simulink model "facsimile_encoding"  (R2016a)
settings: Solver=VariableStepAuto  StartTime=0.0  StopTime=sim_time  RelTol=1e-3
PreLoadFcn:
  | if exist('loadData')
  |     loadData
  | end
StopFcn:
  | if exist('processOutput')
  |     processOutput
  | end
libraries: xbsIndex_r4 x25
settings Model: Creator=hieut  LastModifiedBy=hieut

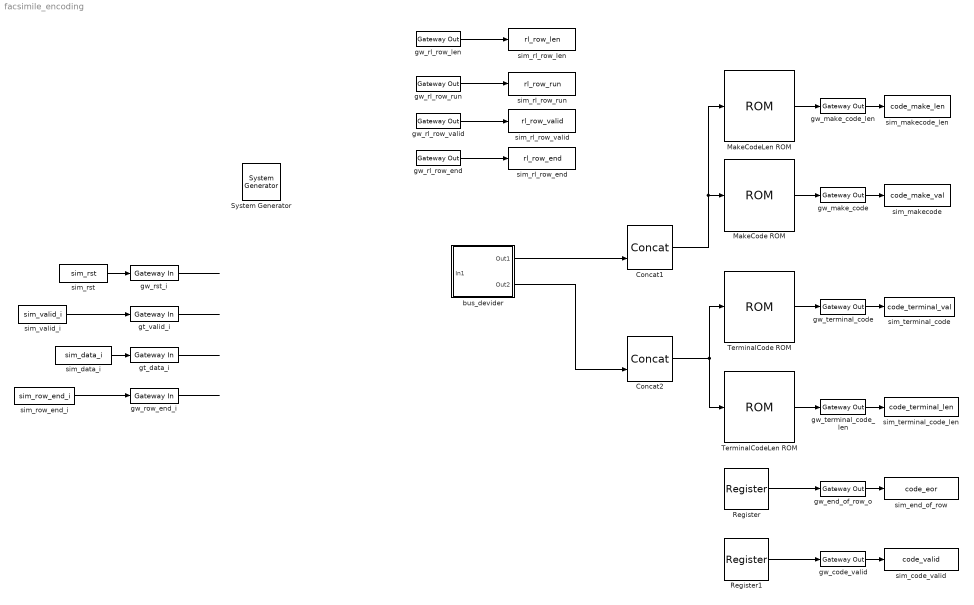
== system facsimile_encoding ==
  " System Generator" : xbsIndex_r4/ System Generator  Tag=genX  xilinxfamily=zynq  part=xc7z010  speed=-1  package=clg400  synthesis_tool=Vivado  clock_wrapper=Clock Enables  directory=./netlist  proj_type=Vivado  Synth_file=Vivado Synthesis Defaults  Impl_file=Vivado Implementation Defaults  testbench=off  simulink_period=1  sysclk_period=10  dcm_input_clock_period=10  incr_netlist=off  trim_vbits=Everywhere in SubSystem  dbl_ovrd=According to Block Masks  core_generation=According to Block Masks  run_coregen=off  deprecated_control=off  eval_field=0  block_type=sysgen
  Concat1 : xbsIndex_r4/Concat  num_inputs=2  dbl_ovrd=off  block_type=concat
  Concat2 : xbsIndex_r4/Concat  num_inputs=2  dbl_ovrd=off  block_type=concat
  MakeCode ROM : xbsIndex_r4/ROM  depth=64  initVector=rom_make_code_values  distributed_mem=Block RAM  rst=off  init_reg=0  en=off  latency=1  gui_display_data_type=Fixed-point  arith_type=Unsigned  n_bits=13  bin_pt=0  preci_type=Single  exp_width=8  frac_width=24  optimize=Area  use_rpm=on  dbl_ovrd=off  block_type=sprom
  MakeCodeLen ROM : xbsIndex_r4/ROM  depth=64  initVector=rom_make_code_lens  distributed_mem=Block RAM  rst=off  init_reg=0  en=off  latency=1  gui_display_data_type=Fixed-point  arith_type=Unsigned  n_bits=13  bin_pt=0  preci_type=Single  exp_width=8  frac_width=24  optimize=Area  use_rpm=on  dbl_ovrd=off  block_type=sprom
  Register : xbsIndex_r4/Register  init=0  rst=off  en=off  dbl_ovrd=off  block_type=register
  Register1 : xbsIndex_r4/Register  init=0  rst=off  en=off  dbl_ovrd=off  block_type=register
  TerminalCode ROM : xbsIndex_r4/ROM  depth=128  initVector=rom_terminal_code_values  distributed_mem=Block RAM  rst=off  init_reg=0  en=off  latency=1  gui_display_data_type=Fixed-point  arith_type=Unsigned  n_bits=13  bin_pt=0  preci_type=Single  exp_width=8  frac_width=24  optimize=Area  use_rpm=on  dbl_ovrd=off  block_type=sprom
  TerminalCodeLen ROM : xbsIndex_r4/ROM  depth=128  initVector=rom_terminal_code_lens  distributed_mem=Block RAM  rst=off  init_reg=0  en=off  latency=1  gui_display_data_type=Fixed-point  arith_type=Unsigned  n_bits=13  bin_pt=0  preci_type=Single  exp_width=8  frac_width=24  optimize=Area  use_rpm=on  dbl_ovrd=off  block_type=sprom
  bus_devider : Subsystem
  gt_data_i : xbsIndex_r4/Gateway In  gui_display_data_type=Boolean  arith_type=Boolean  n_bits=16  bin_pt=14  preci_type=Single  exp_width=8  frac_width=24  rows=1  columns=1  quantization="Round  (unbiased: +/- Inf)"  overflow=Saturate  period=1  UseAsADC=off  ADCChannel='1'  interface=None  automatic_assignment=on  address_offset=hex2dec('00')  intf_name=''  intf_description=''  default_value=0  timing_constraint=None  locs_specified=off  LOCs={}  io_standard={}  inherit_from_input=off  hdl_port=on  dbl_ovrd=off  block_type=gatewayin
  gt_valid_i : xbsIndex_r4/Gateway In  gui_display_data_type=Boolean  arith_type=Boolean  n_bits=16  bin_pt=14  preci_type=Single  exp_width=8  frac_width=24  rows=1  columns=1  quantization="Round  (unbiased: +/- Inf)"  overflow=Saturate  period=1  UseAsADC=off  ADCChannel='1'  interface=None  automatic_assignment=on  address_offset=hex2dec('00')  intf_name=''  intf_description=''  default_value=0  timing_constraint=None  locs_specified=off  LOCs={}  io_standard={}  inherit_from_input=off  hdl_port=on  dbl_ovrd=off  block_type=gatewayin
  gw_code_valid : xbsIndex_r4/Gateway Out  inherit_from_input=off  hdl_port=on  rows=1  columns=1  UseAsDAC=off  DACChannel='1'  interface=None  automatic_assignment=on  address_offset=hex2dec('00')  intf_name=''  intf_description=''  timing_constraint=None  locs_specified=off  LOCs={}  io_standard={}  block_type=gatewayout
  gw_end_of_row_o : xbsIndex_r4/Gateway Out  inherit_from_input=off  hdl_port=on  rows=1  columns=1  UseAsDAC=off  DACChannel='1'  interface=None  automatic_assignment=on  address_offset=hex2dec('00')  intf_name=''  intf_description=''  timing_constraint=None  locs_specified=off  LOCs={}  io_standard={}  block_type=gatewayout
  gw_make_code : xbsIndex_r4/Gateway Out  inherit_from_input=off  hdl_port=on  rows=1  columns=1  UseAsDAC=off  DACChannel='1'  interface=None  automatic_assignment=on  address_offset=hex2dec('00')  intf_name=''  intf_description=''  timing_constraint=None  locs_specified=off  LOCs={}  io_standard={}  block_type=gatewayout
  gw_make_code_len : xbsIndex_r4/Gateway Out  inherit_from_input=off  hdl_port=on  rows=1  columns=1  UseAsDAC=off  DACChannel='1'  interface=None  automatic_assignment=on  address_offset=hex2dec('00')  intf_name=''  intf_description=''  timing_constraint=None  locs_specified=off  LOCs={}  io_standard={}  block_type=gatewayout
  gw_rl_row_end : xbsIndex_r4/Gateway Out  inherit_from_input=off  hdl_port=on  rows=1  columns=1  UseAsDAC=off  DACChannel='1'  interface=None  automatic_assignment=on  address_offset=hex2dec('00')  intf_name=''  intf_description=''  timing_constraint=None  locs_specified=off  LOCs={}  io_standard={}  block_type=gatewayout
  gw_rl_row_len : xbsIndex_r4/Gateway Out  inherit_from_input=off  hdl_port=on  rows=1  columns=1  UseAsDAC=off  DACChannel='1'  interface=None  automatic_assignment=on  address_offset=hex2dec('00')  intf_name=''  intf_description=''  timing_constraint=None  locs_specified=off  LOCs={}  io_standard={}  block_type=gatewayout
  gw_rl_row_run : xbsIndex_r4/Gateway Out  inherit_from_input=off  hdl_port=on  rows=1  columns=1  UseAsDAC=off  DACChannel='1'  interface=None  automatic_assignment=on  address_offset=hex2dec('00')  intf_name=''  intf_description=''  timing_constraint=None  locs_specified=off  LOCs={}  io_standard={}  block_type=gatewayout
  gw_rl_row_valid : xbsIndex_r4/Gateway Out  inherit_from_input=off  hdl_port=on  rows=1  columns=1  UseAsDAC=off  DACChannel='1'  interface=None  automatic_assignment=on  address_offset=hex2dec('00')  intf_name=''  intf_description=''  timing_constraint=None  locs_specified=off  LOCs={}  io_standard={}  block_type=gatewayout
  gw_row_end_i : xbsIndex_r4/Gateway In  gui_display_data_type=Boolean  arith_type=Boolean  n_bits=16  bin_pt=14  preci_type=Single  exp_width=8  frac_width=24  rows=1  columns=1  quantization="Round  (unbiased: +/- Inf)"  overflow=Saturate  period=1  UseAsADC=off  ADCChannel='1'  interface=None  automatic_assignment=on  address_offset=hex2dec('00')  intf_name=''  intf_description=''  default_value=0  timing_constraint=None  locs_specified=off  LOCs={}  io_standard={}  inherit_from_input=off  hdl_port=on  dbl_ovrd=off  block_type=gatewayin
  gw_rst_i : xbsIndex_r4/Gateway In  gui_display_data_type=Boolean  arith_type=Boolean  n_bits=16  bin_pt=14  preci_type=Single  exp_width=8  frac_width=24  rows=1  columns=1  quantization="Round  (unbiased: +/- Inf)"  overflow=Saturate  period=1  UseAsADC=off  ADCChannel='1'  interface=None  automatic_assignment=on  address_offset=hex2dec('00')  intf_name=''  intf_description=''  default_value=0  timing_constraint=None  locs_specified=off  LOCs={}  io_standard={}  inherit_from_input=off  hdl_port=on  dbl_ovrd=off  block_type=gatewayin
  gw_terminal_code : xbsIndex_r4/Gateway Out  inherit_from_input=off  hdl_port=on  rows=1  columns=1  UseAsDAC=off  DACChannel='1'  interface=None  automatic_assignment=on  address_offset=hex2dec('00')  intf_name=''  intf_description=''  timing_constraint=None  locs_specified=off  LOCs={}  io_standard={}  block_type=gatewayout
  gw_terminal_code_len : xbsIndex_r4/Gateway Out  inherit_from_input=off  hdl_port=on  rows=1  columns=1  UseAsDAC=off  DACChannel='1'  interface=None  automatic_assignment=on  address_offset=hex2dec('00')  intf_name=''  intf_description=''  timing_constraint=None  locs_specified=off  LOCs={}  io_standard={}  block_type=gatewayout
  sim_code_valid : ToWorkspace  VariableName=code_valid  SaveFormat=Timeseries  SampleTime=-1
  sim_data_i : FromWorkspace  VariableName=sim_data_i  SampleTime=0
  sim_end_of_row : ToWorkspace  VariableName=code_eor  SaveFormat=Timeseries  SampleTime=-1
  sim_makecode : ToWorkspace  VariableName=code_make_val  SaveFormat=Timeseries  SampleTime=-1
  sim_makecode_len : ToWorkspace  VariableName=code_make_len  SaveFormat=Timeseries  SampleTime=-1
  sim_rl_row_end : ToWorkspace  VariableName=rl_row_end  SaveFormat=Timeseries  SampleTime=-1
  sim_rl_row_len : ToWorkspace  VariableName=rl_row_len  SaveFormat=Timeseries  SampleTime=-1
  sim_rl_row_run : ToWorkspace  VariableName=rl_row_run  SaveFormat=Timeseries  SampleTime=-1
  sim_rl_row_valid : ToWorkspace  VariableName=rl_row_valid  SaveFormat=Timeseries  SampleTime=-1
  sim_row_end_i : FromWorkspace  VariableName=sim_row_end_i  SampleTime=0
  sim_rst : FromWorkspace  VariableName=sim_rst  SampleTime=0
  sim_terminal_code : ToWorkspace  VariableName=code_terminal_val  SaveFormat=Timeseries  SampleTime=-1
  sim_terminal_code_len : ToWorkspace  VariableName=code_terminal_len  SaveFormat=Timeseries  SampleTime=-1
  sim_valid_i : FromWorkspace  VariableName=sim_valid_i  SampleTime=0
  wires:
  sim_rst/1 -> gw_rst_i/1
  sim_valid_i/1 -> gt_valid_i/1
  sim_data_i/1 -> gt_data_i/1
  sim_row_end_i/1 -> gw_row_end_i/1
  ? -> Concat2/1, Concat1/1, gw_rl_row_run/1
  ? -> bus_devider/1(In1), gw_rl_row_len/1
  Concat1/1 -> MakeCodeLen ROM/1, MakeCode ROM/1
  Concat2/1 -> TerminalCodeLen ROM/1, TerminalCode ROM/1
  MakeCodeLen ROM/1 -> gw_make_code_len/1
  MakeCode ROM/1 -> gw_make_code/1
  gt_valid_i/1 -> ?
  gw_rst_i/1 -> ?
  gw_row_end_i/1 -> ?
  gt_data_i/1 -> ?
  gw_end_of_row_o/1 -> sim_end_of_row/1
  gw_terminal_code_len/1 -> sim_terminal_code_len/1
  ? -> Register/1, gw_rl_row_end/1
  Register/1 -> gw_end_of_row_o/1
  TerminalCode ROM/1 -> gw_terminal_code/1
  TerminalCodeLen ROM/1 -> gw_terminal_code_len/1
  gw_make_code_len/1 -> sim_makecode_len/1
  gw_make_code/1 -> sim_makecode/1
  gw_terminal_code/1 -> sim_terminal_code/1
  gw_code_valid/1 -> sim_code_valid/1
  Register1/1 -> gw_code_valid/1
  ? -> Register1/1, gw_rl_row_valid/1
  gw_rl_row_len/1 -> sim_rl_row_len/1
  gw_rl_row_run/1 -> sim_rl_row_run/1
  gw_rl_row_valid/1 -> sim_rl_row_valid/1
  gw_rl_row_end/1 -> sim_rl_row_end/1
  bus_devider/1(Out1) -> Concat1/2
  bus_devider/2(Out2) -> Concat2/2

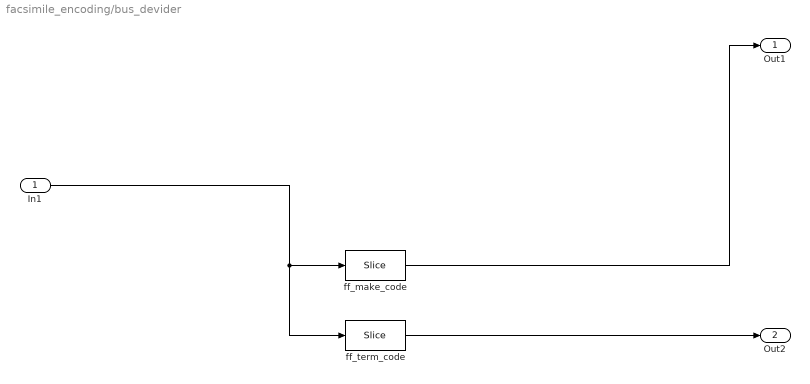
== system facsimile_encoding/bus_devider ==
  In1 : Inport
  ff_make_code : xbsIndex_r4/Slice  nbits=5  boolean_output=off  mode=Two Bit Locations  bit1=10  base1=LSB of Input  bit0=6  base0=LSB of Input  dbl_ovrd=off  block_type=slice
  ff_term_code : xbsIndex_r4/Slice  nbits=6  boolean_output=off  mode=Two Bit Locations  bit1=5  base1=LSB of Input  bit0=0  base0=LSB of Input  dbl_ovrd=off  block_type=slice
  Out1 : Outport
  Out2 : Outport  Port=2
  wires:
  In1/1 -> ff_term_code/1, ff_make_code/1
  ff_make_code/1 -> Out1/1
  ff_term_code/1 -> Out2/1
